simulink model "sampleModel653"  (R2023a)
settings: Solver=VariableStepAuto  StartTime=0.0  StopTime=10.0  RelTol=1e-3
undefined symbols (not defined in the file): DiscIntNeverNeededParam, magnitude, Newton, Raphson
libraries: simulink x238, slpidlib x68
(part 2 of 11)

== system sampleModel653/cfblk135 ==
  cfblk1 : Inport
  cfblk10 : Inport  Port=2
  cfblk{3,11..17} (8 alike) : Delay  SampleTime=1
  cfblk4 : slpidlib/PID Controller (2DOF)  Controller=PID  Form=Parallel  TimeDomain=Discrete-time  UseExternalTs=off  SampleTime=1  IntegratorMethod=Forward Euler  FilterMethod=Forward Euler  ControllerParametersSource=internal  P=1  I=1  UseKiTs=off  D=0  N=100  UseFilter=on  b=1  c=1  TunerSelectOption=Transfer Function Based (PID Tuner App)  InitialConditionSource=internal  InitialConditionForIntegrator=0  InitialConditionForFilter=0  DifferentiatorICPrevScaledInput=0  ExternalReset=none  TrackingMode=off  Kt=1  LimitOutput=off  SatLimitsSource=internal  UpperSaturationLimit=inf  LowerSaturationLimit=-inf  LinearizeAsGain=off  AntiWindupMode=none  Kb=1  LimitIntegrator=off  UpperIntegratorSaturationLimit=inf  LowerIntegratorSaturationLimit=-inf  POutMin=[]  POutMax=[]  IOutMin=[]  IOutMax=[]  DOutMin=[]  DOutMax=[]  NOutMin=[]  NOutMax=[]  bOutMin=[]  bOutMax=[]  cOutMin=[]  cOutMax=[]  SumOutMin=[]  SumOutMax=[]  SaturationOutMin=[]  SaturationOutMax=[]  PParamMin=[]  PParamMax=[]  IParamMin=[]  IParamMax=[]  DParamMin=[]  DParamMax=[]  NParamMin=[]  NParamMax=[]  bParamMin=[]  bParamMax=[]  cParamMin=[]  cParamMax=[]  KbParamMin=[]  KbParamMax=[]  KtParamMin=[]  KtParamMax=[]  KbOutMin=[]  KbOutMax=[]  KtOutMin=[]  KtOutMax=[]  IntegratorOutMin=[]  IntegratorOutMax=[]  FilterOutMin=[]  FilterOutMax=[]  SumI1OutMin=[]  SumI1OutMax=[]  SumI2OutMin=[]  SumI2OutMax=[]  SumI3OutMin=[]  SumI3OutMax=[]  SumI4OutMin=[]  SumI4OutMax=[]  SumDOutMin=[]  SumDOutMax=[]  Sum1OutMin=[]  Sum1OutMax=[]  Sum2OutMin=[]  Sum2OutMax=[]  Sum3OutMin=[]  Sum3OutMax=[]  DifferentiatorOutMin=[]  DifferentiatorOutMax=[]  FilterDiffOutCoefMin=[]  FilterDiffOutCoefMax=[]  ReciprocalOutMin=[]  ReciprocalOutMax=[]  SumDenOutMin=[]  SumDenOutMax=[]  SumNumOutMin=[]  SumNumOutMax=[]  DivideOutMin=[]  DivideOutMax=[]  UdiffTsProdOutMin=[]  UdiffTsProdOutMax=[]  NTsProdOutMin=[]  NTsProdOutMax=[]  UintegralTsProdOutMin=[]  UintegralTsProdOutMax=[]  UngainTsProdOutMin=[]  UngainTsProdOutMax=[]  ClampingZeroOutDataTypeStr=Inherit: Inherit via back propagation  ClampingZeroOutMin=[]  ClampingZeroOutMax=[]  FilterDenConstantOutDataTypeStr=Inherit: Inherit via back propagation  FilterDenConstantOutMin=[]  FilterDenConstantOutMax=[]  PCopyOutDataTypeStr=Inherit: Inherit via back propagation  PCopyOutMin=[]  PCopyOutMax=[]  NCopyOutDataTypeStr=Inherit: Inherit via back propagation  NCopyOutMin=[]  NCopyOutMax=[]  IntegratorContinuousStateAttributes=''  IntegratorStateMustResolveToSignalObject=off  IntegratorRTWStateStorageClass=Auto  FilterContinuousStateAttributes=''  FilterStateMustResolveToSignalObject=off  FilterRTWStateStorageClass=Auto  ParallelPVariant=InternalParameters  IdealPVariant=Disabled  IVariant=InternalParameters  DVariant=InternalParameters  bVariant=InternalParameters  cVariant=InternalParameters  IntegratorVariant=Discrete  SatVariant=Disabled  AWVariant=Passthrough  PCopyVariant=Disabled  TRVariant=Disabled  FdbkBlocksVariant=Forward  IdealPFdbkVariant=Disabled  SatFdbkVariant=Disabled  DerivativeFilterVariant=ForwardEulerFilter  NVariant=InternalParameters  NCopyVariant=Disabled  FilterICVariant=InternalICsFilter  IntegratorICVariant=InternalICs  ExternalResetVariant=Disabled  TRSumVariant=Passthrough  SumFdbkVariant=Disabled  SumVariant=Sum_PID  TsampFilterVariant=InternalTs  TsampNgainVariant=Passthrough  TsampIntegralVariant=Disabled_SignalSpec  ExternalSaturationOutDataTypeStr=Inherit: Same as second input
      settings: LibrarySourceBlock=simulink/Discrete/Discrete PID Controller (2DOF)
  cfblk5 : simulink/Discrete/Transfer Fcn Lead or Lag  PoleZ=0.95  ZeroZ=0.75  ICPrevOutput=0.0  ICPrevInput=0.0  DoSatur=off
  cfblk6 : MinMax  Inputs=3
  cfblk7 : Subsystem
  cfblk8 : Subsystem
  cfblk9 : Subsystem
  cfblk2 : Outport
  wires:
  cfblk9/1(cfblk2) -> cfblk2/1
  cfblk9/2(cfblk14) -> cfblk3/1, cfblk11/1
  cfblk10/1 -> cfblk8/2(cfblk11), cfblk9/2(cfblk12), cfblk6/3
  cfblk8/1(cfblk2) -> cfblk9/1(cfblk1), cfblk6/2
  cfblk1/1 -> cfblk4/1
  cfblk7/1(cfblk2) -> cfblk5/1, cfblk17/1
  cfblk5/1 -> cfblk15/1, cfblk16/1
  cfblk6/1 -> cfblk7/3(cfblk7), cfblk12/1, cfblk13/1, cfblk14/1
  cfblk4/1 -> cfblk8/4(cfblk13)
  cfblk3/1 -> cfblk6/1, cfblk7/2(cfblk6)
  cfblk11/1 -> cfblk8/1(cfblk1)
  cfblk12/1 -> cfblk8/3(cfblk12)
  cfblk13/1 -> cfblk9/3(cfblk13)
  cfblk14/1 -> cfblk8/5(cfblk14)
  cfblk15/1 -> cfblk4/2
  cfblk16/1 -> cfblk7/1(cfblk1)
  cfblk17/1 -> cfblk8/6(cfblk15)

== system sampleModel653/cfblk136 ==
  cfblk1 : Inport
  cfblk3 : DiscreteIntegrator  ICPrevOutput=DiscIntNeverNeededParam  ICPrevScaledInput=DiscIntNeverNeededParam
  cfblk4 : Trigonometry
  cfblk5 : Squeeze
  cfblk6 : Constant  Value=[-159954110.275562]  SampleTime=1
  cfblk7 : Subsystem
  cfblk8 : Delay  SampleTime=1
  cfblk2 : Outport
  wires:
  cfblk6/1 -> cfblk5/1
  cfblk3/1 -> cfblk2/1, cfblk8/1
  cfblk7/1(cfblk2) -> cfblk3/1
  cfblk1/1 -> cfblk7/1(cfblk1)
  cfblk5/1 -> cfblk4/1
  cfblk4/1 -> cfblk7/2(cfblk13)
  cfblk8/1 -> cfblk7/3(cfblk14)

== system sampleModel653/cfblk137 ==
  cfblk1 : Inport
  cfblk13 : Inport  Port=2
  cfblk10 : Subsystem
  cfblk11 : Subsystem
  cfblk12 : Subsystem
  cfblk15 : Delay  SampleTime=1
  cfblk16 : Delay  SampleTime=1
  cfblk17 : Delay  SampleTime=1
  cfblk3 : DiscreteTransferFcn  SampleTime=1
  cfblk4 : DiscreteStateSpace
  cfblk5 : Signum
  cfblk6 : simulink/Math Operations/MinMax Running Resettable  Function=min  vinit=0.0
  cfblk7 : Reshape
  cfblk8 : Constant  Value=[-21079559.337521]  SampleTime=1
  cfblk9 : Subsystem
  cfblk2 : Outport
  cfblk14 : Outport  Port=2
  wires:
  cfblk4/1 -> cfblk10/1(cfblk1)
  cfblk5/1 -> cfblk14/1, cfblk9/2(cfblk7)
  cfblk8/1 -> cfblk10/2(cfblk12), cfblk9/3(cfblk8)
  cfblk9/1(cfblk2) -> cfblk4/1
  cfblk7/1 -> cfblk12/1(cfblk1)
  cfblk6/1 -> cfblk5/1
  cfblk3/1 -> cfblk2/1
  cfblk1/1 -> cfblk7/1, cfblk9/4(cfblk9)
  cfblk11/1(cfblk2) -> cfblk6/2
  cfblk13/1 -> cfblk12/2(cfblk6)
  cfblk10/2(cfblk13) -> cfblk16/1, cfblk17/1
  cfblk12/1(cfblk2) -> cfblk3/1
  cfblk12/2(cfblk7) -> cfblk11/1(cfblk1)
  cfblk10/1(cfblk2) -> cfblk15/1
  cfblk15/1 -> cfblk6/1
  cfblk16/1 -> cfblk9/1(cfblk1)
  cfblk17/1 -> cfblk11/2(cfblk8)

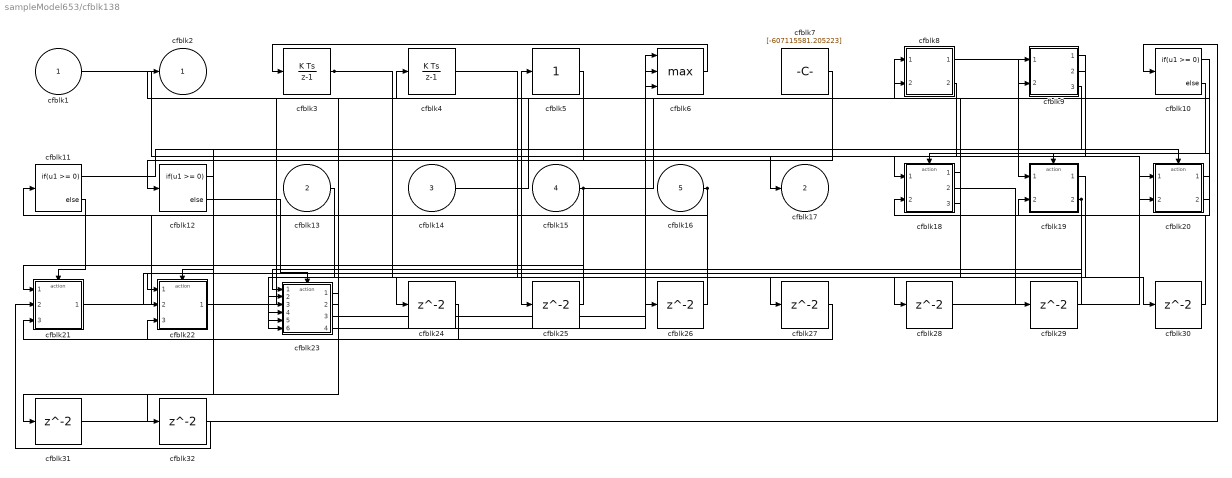
== system sampleModel653/cfblk138 ==
  cfblk1 : Inport
  cfblk13 : Inport  Port=2
  cfblk14 : Inport  Port=3
  cfblk15 : Inport  Port=4
  cfblk16 : Inport  Port=5
  cfblk10 : If  IfExpression=u1 >= 0  SampleTime=1
  cfblk11 : If  IfExpression=u1 >= 0  SampleTime=1
  cfblk12 : If  IfExpression=u1 >= 0  SampleTime=1
  cfblk18 : Subsystem  TreatAsAtomicUnit=on
  cfblk19 : Subsystem  TreatAsAtomicUnit=on
  cfblk20 : Subsystem  TreatAsAtomicUnit=on
  cfblk21 : Subsystem  TreatAsAtomicUnit=on
  cfblk22 : Subsystem  TreatAsAtomicUnit=on
  cfblk23 : Subsystem  TreatAsAtomicUnit=on
  cfblk{24..32} (9 alike) : Delay  SampleTime=1
  cfblk3 : DiscreteIntegrator  ICPrevOutput=DiscIntNeverNeededParam  ICPrevScaledInput=DiscIntNeverNeededParam
  cfblk4 : DiscreteIntegrator  ICPrevOutput=DiscIntNeverNeededParam  ICPrevScaledInput=DiscIntNeverNeededParam
  cfblk5 : simulink/Math Operations/Slider Gain  gain=1  low=0  high=2
  cfblk6 : MinMax  Function=max  Inputs=3
  cfblk7 : Constant  Value=[-607115581.205223]  SampleTime=1
  cfblk8 : Subsystem
  cfblk9 : Subsystem
  cfblk2 : Outport
  cfblk17 : Outport  Port=2
  wires:
  cfblk9/1(cfblk2) -> cfblk18/1(cfblk1)
  cfblk3/1 -> cfblk26/1, cfblk27/1
  cfblk15/1 -> cfblk8/1(cfblk1), cfblk23/4(cfblk12), cfblk9/2(cfblk12)
  cfblk7/1 -> cfblk12/1
  cfblk21/1(cfblk2) -> cfblk5/1
  cfblk1/1 -> cfblk20/2(cfblk13)
  cfblk22/1(cfblk2) -> cfblk6/1
  cfblk9/2(cfblk13) -> cfblk17/1
  cfblk18/3(cfblk9) -> cfblk4/1
  cfblk16/1 -> cfblk23/2(cfblk10), cfblk23/5(cfblk13)
  cfblk6/1 -> cfblk3/1
  cfblk14/1 -> cfblk8/2(cfblk7)
  cfblk8/1(cfblk2) -> cfblk19/1(cfblk1)
  cfblk8/2(cfblk8) -> cfblk22/1(cfblk1)
  cfblk20/1(cfblk2) -> cfblk19/2(cfblk12)
  cfblk13/1 -> cfblk23/3(cfblk11)
  cfblk19/2(cfblk13) -> cfblk22/2(cfblk7), cfblk23/6(cfblk14)
  cfblk20/2(cfblk14) -> cfblk9/1(cfblk1)
  cfblk23/2(cfblk15) -> cfblk2/1
  cfblk23/3(cfblk16) -> cfblk6/2
  cfblk23/4(cfblk17) -> cfblk6/3
  cfblk10/1 -> cfblk18/Action
  cfblk10/2 -> cfblk19/Action
  cfblk11/1 -> cfblk20/Action
  cfblk11/2 -> cfblk21/Action
  cfblk12/1 -> cfblk22/Action
  cfblk12/2 -> cfblk23/Action
  cfblk19/1(cfblk2) -> cfblk24/1
  cfblk24/1 -> cfblk21/3(cfblk12)
  cfblk5/1 -> cfblk25/1
  cfblk25/1 -> cfblk21/1(cfblk1)
  cfblk26/1 -> cfblk11/1
  cfblk27/1 -> cfblk22/3(cfblk8)
  cfblk18/1(cfblk2) -> cfblk28/1
  cfblk28/1 -> cfblk20/1(cfblk1)
  cfblk18/2(cfblk8) -> cfblk29/1
  cfblk29/1 -> cfblk23/1(cfblk1)
  cfblk4/1 -> cfblk30/1
  cfblk30/1 -> cfblk18/2(cfblk7)
  cfblk23/1(cfblk2) -> cfblk31/1
  cfblk31/1 -> cfblk10/1
  cfblk9/3(cfblk14) -> cfblk32/1
  cfblk32/1 -> cfblk21/2(cfblk11)

== system sampleModel653/cfblk139 ==
  cfblk1 : Inport
  cfblk14 : Inport  Port=2
  cfblk15 : Inport  Port=3
  cfblk10 : Subsystem
  cfblk11 : Subsystem
  cfblk12 : Subsystem
  cfblk13 : Subsystem
  cfblk{17..21} (5 alike) : Delay  SampleTime=1
  cfblk3 : PropagationDelay  SampleTime=1
  cfblk4 : DiscreteZeroPole  Poles=[0 0.5]  Gain=1
  cfblk5 : Signum
  cfblk6 : Assignment  DiagnosticForDimensions=Warning  IndexOptions=Index vector (dialog)  Indices=1  OutputSizes=1
  cfblk7 : PermuteDimensions
  cfblk8 : Abs  SaturateOnIntegerOverflow=off
  cfblk9 : Sum  Inputs=+-
  cfblk2 : Outport
  cfblk16 : Outport  Port=2
  wires:
  cfblk12/1(cfblk2) -> cfblk7/1
  cfblk15/1 -> cfblk9/1, cfblk11/6(cfblk16)
  cfblk12/2(cfblk11) -> cfblk11/1(cfblk1)
  cfblk9/1 -> cfblk2/1
  cfblk11/1(cfblk2) -> cfblk3/1
  cfblk1/1 -> cfblk5/1
  cfblk4/1 -> cfblk20/1, cfblk21/1
  cfblk3/1 -> cfblk4/1
  cfblk7/1 -> cfblk18/1, cfblk19/1
  cfblk10/1(cfblk2) -> cfblk8/1
  cfblk12/3(cfblk12) -> cfblk3/2
  cfblk5/1 -> cfblk6/2, cfblk11/3(cfblk13)
  cfblk12/4(cfblk13) -> cfblk9/2
  cfblk10/2(cfblk8) -> cfblk13/2(cfblk6)
  cfblk14/1 -> cfblk10/1(cfblk1)
  cfblk13/1(cfblk2) -> cfblk12/1(cfblk1)
  cfblk6/1 -> cfblk10/2(cfblk7), cfblk11/4(cfblk14)
  cfblk10/3(cfblk9) -> cfblk16/1, cfblk13/3(cfblk7), cfblk13/4(cfblk8)
  cfblk8/1 -> cfblk17/1
  cfblk17/1 -> cfblk6/1
  cfblk18/1 -> cfblk13/1(cfblk1)
  cfblk19/1 -> cfblk12/2(cfblk10)
  cfblk20/1 -> cfblk11/2(cfblk12)
  cfblk21/1 -> cfblk11/5(cfblk15)

== system sampleModel653/cfblk140 ==
  cfblk1 : Inport
  cfblk7 : Inport  Port=2
  cfblk8 : Inport  Port=3
  cfblk9 : Inport  Port=4
  cfblk10 : Inport  Port=5
  cfblk11 : Delay  SampleTime=1
  cfblk3 : PermuteDimensions
  cfblk4 : Subsystem
  cfblk5 : Subsystem
  cfblk6 : Subsystem
  cfblk2 : Outport
  wires:
  cfblk10/1 -> cfblk4/2(cfblk11), cfblk6/5(cfblk7)
  cfblk8/1 -> cfblk2/1
  cfblk7/1 -> cfblk5/1(cfblk1), cfblk6/2(cfblk4)
  cfblk9/1 -> cfblk4/3(cfblk12)
  cfblk1/1 -> cfblk4/4(cfblk13), cfblk6/3(cfblk5)
  cfblk5/1(cfblk2) -> cfblk3/1
  cfblk6/1(cfblk2) -> cfblk5/2(cfblk7)
  cfblk4/1(cfblk2) -> cfblk5/3(cfblk8)
  cfblk4/2(cfblk14) -> cfblk6/1(cfblk1), cfblk6/4(cfblk6)
  cfblk3/1 -> cfblk11/1
  cfblk11/1 -> cfblk4/1(cfblk1)

== system sampleModel653/cfblk141 ==
  cfblk1 : Inport
  cfblk5 : Inport  Port=2
  cfblk3 : DiscreteIntegrator  ICPrevOutput=DiscIntNeverNeededParam  ICPrevScaledInput=DiscIntNeverNeededParam
  cfblk4 : DotProduct  OutDataTypeStr=Inherit: Inherit via internal rule
  cfblk2 : Outport
  cfblk6 : Outport  Port=2
  cfblk7 : Outport  Port=3
  wires:
  cfblk5/1 -> cfblk4/1
  cfblk4/1 -> cfblk6/1, cfblk3/1
  cfblk3/1 -> cfblk2/1, cfblk7/1
  cfblk1/1 -> cfblk4/2

== system sampleModel653/cfblk142 ==
  cfblk1 : Inport
  cfblk15 : Inport  Port=2
  cfblk10 : Subsystem
  cfblk11 : Subsystem
  cfblk12 : Subsystem
  cfblk13 : Subsystem
  cfblk14 : Subsystem
  cfblk{17..21} (5 alike) : Delay  SampleTime=1
  cfblk3 : slpidlib/PID Controller (2DOF)  Controller=PID  Form=Parallel  TimeDomain=Discrete-time  UseExternalTs=off  SampleTime=1  IntegratorMethod=Forward Euler  FilterMethod=Forward Euler  ControllerParametersSource=internal  P=1  I=1  UseKiTs=off  D=0  N=100  UseFilter=on  b=1  c=1  TunerSelectOption=Transfer Function Based (PID Tuner App)  InitialConditionSource=internal  InitialConditionForIntegrator=0  InitialConditionForFilter=0  DifferentiatorICPrevScaledInput=0  ExternalReset=none  TrackingMode=off  Kt=1  LimitOutput=off  SatLimitsSource=internal  UpperSaturationLimit=inf  LowerSaturationLimit=-inf  LinearizeAsGain=off  AntiWindupMode=none  Kb=1  LimitIntegrator=off  UpperIntegratorSaturationLimit=inf  LowerIntegratorSaturationLimit=-inf  POutMin=[]  POutMax=[]  IOutMin=[]  IOutMax=[]  DOutMin=[]  DOutMax=[]  NOutMin=[]  NOutMax=[]  bOutMin=[]  bOutMax=[]  cOutMin=[]  cOutMax=[]  SumOutMin=[]  SumOutMax=[]  SaturationOutMin=[]  SaturationOutMax=[]  PParamMin=[]  PParamMax=[]  IParamMin=[]  IParamMax=[]  DParamMin=[]  DParamMax=[]  NParamMin=[]  NParamMax=[]  bParamMin=[]  bParamMax=[]  cParamMin=[]  cParamMax=[]  KbParamMin=[]  KbParamMax=[]  KtParamMin=[]  KtParamMax=[]  KbOutMin=[]  KbOutMax=[]  KtOutMin=[]  KtOutMax=[]  IntegratorOutMin=[]  IntegratorOutMax=[]  FilterOutMin=[]  FilterOutMax=[]  SumI1OutMin=[]  SumI1OutMax=[]  SumI2OutMin=[]  SumI2OutMax=[]  SumI3OutMin=[]  SumI3OutMax=[]  SumI4OutMin=[]  SumI4OutMax=[]  SumDOutMin=[]  SumDOutMax=[]  Sum1OutMin=[]  Sum1OutMax=[]  Sum2OutMin=[]  Sum2OutMax=[]  Sum3OutMin=[]  Sum3OutMax=[]  DifferentiatorOutMin=[]  DifferentiatorOutMax=[]  FilterDiffOutCoefMin=[]  FilterDiffOutCoefMax=[]  ReciprocalOutMin=[]  ReciprocalOutMax=[]  SumDenOutMin=[]  SumDenOutMax=[]  SumNumOutMin=[]  SumNumOutMax=[]  DivideOutMin=[]  DivideOutMax=[]  UdiffTsProdOutMin=[]  UdiffTsProdOutMax=[]  NTsProdOutMin=[]  NTsProdOutMax=[]  UintegralTsProdOutMin=[]  UintegralTsProdOutMax=[]  UngainTsProdOutMin=[]  UngainTsProdOutMax=[]  ClampingZeroOutDataTypeStr=Inherit: Inherit via back propagation  ClampingZeroOutMin=[]  ClampingZeroOutMax=[]  FilterDenConstantOutDataTypeStr=Inherit: Inherit via back propagation  FilterDenConstantOutMin=[]  FilterDenConstantOutMax=[]  PCopyOutDataTypeStr=Inherit: Inherit via back propagation  PCopyOutMin=[]  PCopyOutMax=[]  NCopyOutDataTypeStr=Inherit: Inherit via back propagation  NCopyOutMin=[]  NCopyOutMax=[]  IntegratorContinuousStateAttributes=''  IntegratorStateMustResolveToSignalObject=off  IntegratorRTWStateStorageClass=Auto  FilterContinuousStateAttributes=''  FilterStateMustResolveToSignalObject=off  FilterRTWStateStorageClass=Auto  ParallelPVariant=InternalParameters  IdealPVariant=Disabled  IVariant=InternalParameters  DVariant=InternalParameters  bVariant=InternalParameters  cVariant=InternalParameters  IntegratorVariant=Discrete  SatVariant=Disabled  AWVariant=Passthrough  PCopyVariant=Disabled  TRVariant=Disabled  FdbkBlocksVariant=Forward  IdealPFdbkVariant=Disabled  SatFdbkVariant=Disabled  DerivativeFilterVariant=ForwardEulerFilter  NVariant=InternalParameters  NCopyVariant=Disabled  FilterICVariant=InternalICsFilter  IntegratorICVariant=InternalICs  ExternalResetVariant=Disabled  TRSumVariant=Passthrough  SumFdbkVariant=Disabled  SumVariant=Sum_PID  TsampFilterVariant=InternalTs  TsampNgainVariant=Passthrough  TsampIntegralVariant=Disabled_SignalSpec  ExternalSaturationOutDataTypeStr=Inherit: Same as second input
      settings: LibrarySourceBlock=simulink/Discrete/Discrete PID Controller (2DOF)
  cfblk4 : DiscreteTransferFcn  SampleTime=1
  cfblk5 : Sqrt  Operator=rSqrt  AlgorithmType=Newton-Raphson
  cfblk6 : Reshape
  cfblk7 : Squeeze
  cfblk8 : Constant  Value=[687668237.338755]  SampleTime=1
  cfblk9 : Constant  Value=[-134938551.246694]  SampleTime=1
  cfblk2 : Outport
  cfblk16 : Outport  Port=2
  wires:
  cfblk11/1(cfblk2) -> cfblk5/1
  cfblk6/1 -> cfblk16/1
  cfblk15/1 -> cfblk3/1, cfblk13/5(cfblk12)
  cfblk14/1(cfblk2) -> cfblk11/1(cfblk1), cfblk11/3(cfblk12), cfblk18/1, cfblk19/1
  cfblk7/1 -> cfblk3/2
  cfblk9/1 -> cfblk14/1(cfblk1), cfblk12/5(cfblk11)
  cfblk13/1(cfblk2) -> cfblk2/1
  cfblk3/1 -> cfblk14/2(cfblk13), cfblk20/1
  cfblk1/1 -> cfblk6/1, cfblk13/3(cfblk10)
  cfblk8/1 -> cfblk13/2(cfblk9)
  cfblk13/2(cfblk13) -> cfblk10/1(cfblk1), cfblk11/4(cfblk13)
  cfblk10/1(cfblk2) -> cfblk12/1(cfblk1)
  cfblk12/1(cfblk2) -> cfblk14/3(cfblk14)
  cfblk10/2(cfblk11) -> cfblk12/2(cfblk8), cfblk14/5(cfblk16)
  cfblk12/2(cfblk12) -> cfblk14/4(cfblk15)
  cfblk12/3(cfblk13) -> cfblk11/2(cfblk11)
  cfblk12/4(cfblk14) -> cfblk4/1, cfblk21/1
  cfblk4/1 -> cfblk7/1
  cfblk5/1 -> cfblk17/1
  cfblk17/1 -> cfblk13/1(cfblk1)
  cfblk18/1 -> cfblk10/2(cfblk10)
  cfblk19/1 -> cfblk12/3(cfblk9)
  cfblk20/1 -> cfblk12/4(cfblk10)
  cfblk21/1 -> cfblk13/4(cfblk11)

== system sampleModel653/cfblk143 ==
  cfblk1 : Inport
  cfblk10 : Subsystem
  cfblk11 : Delay  SampleTime=1
  cfblk12 : Delay  SampleTime=1
  cfblk13 : Delay  SampleTime=1
  cfblk3 : simulink/Discrete/Difference  ICPrevInput=0.0  OutMin=[]  OutMax=[]  OutDataTypeStr=Inherit: Inherit via back propagation  OutDataType=fixdt(1, 16)  OutScaling=2^-10  DoSatur=off
  cfblk4 : simulink/Discrete/Transfer Fcn First Order  PoleZ=0.95  ICPrevOutput=0.0  DoSatur=off
  cfblk5 : simulink/Discrete/Difference  ICPrevInput=0.0  OutMin=[]  OutMax=[]  OutDataTypeStr=Inherit: Inherit via back propagation  OutDataType=fixdt(1, 16)  OutScaling=2^-10  DoSatur=off
  cfblk6 : Gain  Gain=[-693180009.173398]
  cfblk7 : UnaryMinus
  cfblk8 : Subsystem
  cfblk9 : Subsystem
  cfblk2 : Outport
  wires:
  cfblk4/1 -> cfblk10/1(cfblk1)
  cfblk3/1 -> cfblk7/1
  cfblk7/1 -> cfblk5/1
  cfblk6/1 -> cfblk2/1, cfblk8/2(cfblk8)
  cfblk10/1(cfblk2) -> cfblk9/1(cfblk1)
  cfblk1/1 -> cfblk6/1
  cfblk8/1(cfblk2) -> cfblk3/1
  cfblk5/1 -> cfblk11/1
  cfblk11/1 -> cfblk8/1(cfblk1)
  cfblk9/1(cfblk2) -> cfblk12/1
  cfblk12/1 -> cfblk4/1
  cfblk9/2(cfblk7) -> cfblk13/1
  cfblk13/1 -> cfblk10/2(cfblk8)

== system sampleModel653/cfblk144 ==
  cfblk1 : Inport
  cfblk7 : Inport  Port=2
  cfblk3 : ComplexToRealImag
  cfblk4 : Sqrt
  cfblk5 : Subsystem
  cfblk6 : Subsystem
  cfblk9 : Delay  SampleTime=1
  cfblk2 : Outport
  cfblk8 : Outport  Port=2
  wires:
  cfblk3/1 -> cfblk6/1(cfblk1)
  cfblk5/1(cfblk2) -> cfblk6/2(cfblk8), cfblk9/1
  cfblk4/1 -> cfblk5/1(cfblk1)
  cfblk3/2 -> cfblk4/1, cfblk5/3(cfblk7)
  cfblk7/1 -> cfblk5/2(cfblk6)
  cfblk1/1 -> cfblk8/1
  cfblk6/1(cfblk2) -> cfblk2/1
  cfblk9/1 -> cfblk3/1

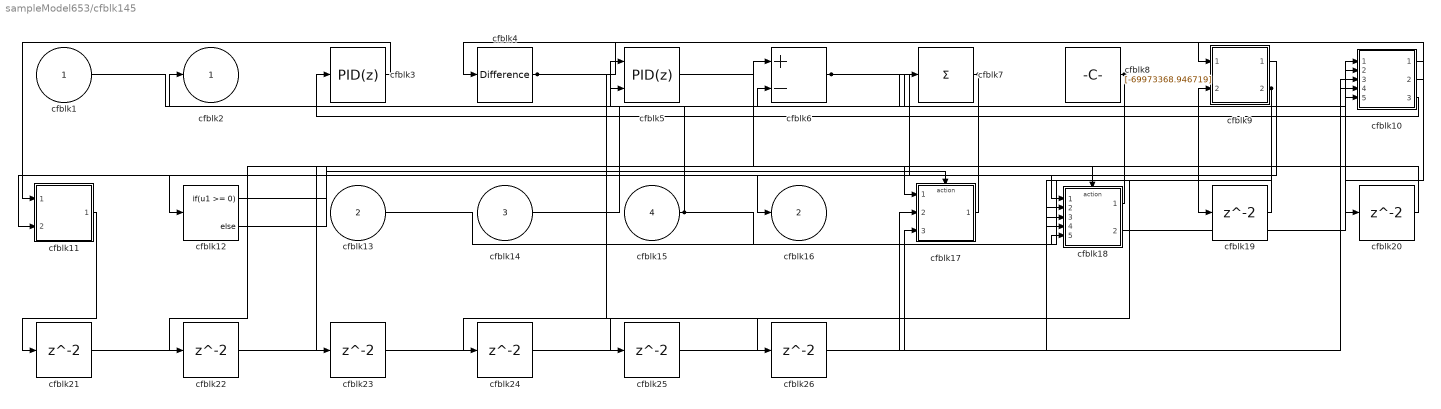
== system sampleModel653/cfblk145 ==
  cfblk1 : Inport
  cfblk13 : Inport  Port=2
  cfblk14 : Inport  Port=3
  cfblk15 : Inport  Port=4
  cfblk10 : Subsystem
  cfblk11 : Subsystem
  cfblk12 : If  IfExpression=u1 >= 0  SampleTime=1
  cfblk17 : Subsystem  TreatAsAtomicUnit=on
  cfblk18 : Subsystem  TreatAsAtomicUnit=on
  cfblk{19..26} (8 alike) : Delay  SampleTime=1
  cfblk3 : slpidlib/PID Controller  Controller=PID  Form=Parallel  TimeDomain=Discrete-time  UseExternalTs=off  SampleTime=1  IntegratorMethod=Forward Euler  FilterMethod=Forward Euler  ControllerParametersSource=internal  P=1  I=1  UseKiTs=off  D=0  N=100  UseFilter=on  TunerSelectOption=Transfer Function Based (PID Tuner App)  InitialConditionSource=internal  InitialConditionForIntegrator=0  InitialConditionForFilter=0  DifferentiatorICPrevScaledInput=0  ExternalReset=none  TrackingMode=off  Kt=1  LimitOutput=off  SatLimitsSource=internal  UpperSaturationLimit=inf  LowerSaturationLimit=-inf  LinearizeAsGain=off  AntiWindupMode=none  Kb=1  LimitIntegrator=off  UpperIntegratorSaturationLimit=inf  LowerIntegratorSaturationLimit=-inf  POutMin=[]  POutMax=[]  IOutMin=[]  IOutMax=[]  DOutMin=[]  DOutMax=[]  NOutMin=[]  NOutMax=[]  SumOutMin=[]  SumOutMax=[]  SaturationOutMin=[]  SaturationOutMax=[]  PParamMin=[]  PParamMax=[]  IParamMin=[]  IParamMax=[]  DParamMin=[]  DParamMax=[]  NParamMin=[]  NParamMax=[]  KbParamMin=[]  KbParamMax=[]  KtParamMin=[]  KtParamMax=[]  KbOutMin=[]  KbOutMax=[]  KtOutMin=[]  KtOutMax=[]  IntegratorOutMin=[]  IntegratorOutMax=[]  FilterOutMin=[]  FilterOutMax=[]  SumI1OutMin=[]  SumI1OutMax=[]  SumI2OutMin=[]  SumI2OutMax=[]  SumI3OutMin=[]  SumI3OutMax=[]  SumI4OutMin=[]  SumI4OutMax=[]  SumDOutMin=[]  SumDOutMax=[]  DifferentiatorOutMin=[]  DifferentiatorOutMax=[]  FilterDiffOutCoefMin=[]  FilterDiffOutCoefMax=[]  ReciprocalOutMin=[]  ReciprocalOutMax=[]  SumDenOutMin=[]  SumDenOutMax=[]  SumNumOutMin=[]  SumNumOutMax=[]  DivideOutMin=[]  DivideOutMax=[]  UdiffTsProdOutMin=[]  UdiffTsProdOutMax=[]  NTsProdOutMin=[]  NTsProdOutMax=[]  UintegralTsProdOutMin=[]  UintegralTsProdOutMax=[]  UngainTsProdOutMin=[]  UngainTsProdOutMax=[]  ClampingZeroOutDataTypeStr=Inherit: Inherit via back propagation  ClampingZeroOutMin=[]  ClampingZeroOutMax=[]  FilterDenConstantOutDataTypeStr=Inherit: Inherit via back propagation  FilterDenConstantOutMin=[]  FilterDenConstantOutMax=[]  PCopyOutDataTypeStr=Inherit: Inherit via back propagation  PCopyOutMin=[]  PCopyOutMax=[]  NCopyOutDataTypeStr=Inherit: Inherit via back propagation  NCopyOutMin=[]  NCopyOutMax=[]  IntegratorContinuousStateAttributes=''  IntegratorStateMustResolveToSignalObject=off  IntegratorRTWStateStorageClass=Auto  FilterContinuousStateAttributes=''  FilterStateMustResolveToSignalObject=off  FilterRTWStateStorageClass=Auto  ParallelPVariant=InternalParameters  IdealPVariant=Disabled  IVariant=InternalParameters  DVariant=InternalParameters  IntegratorVariant=Discrete  SatVariant=Disabled  AWVariant=Passthrough  PCopyVariant=Disabled  TRVariant=Disabled  FdbkBlocksVariant=Forward  IdealPFdbkVariant=Disabled  SatFdbkVariant=Disabled  DerivativeFilterVariant=ForwardEulerFilter  NVariant=InternalParameters  NCopyVariant=Disabled  FilterICVariant=InternalICsFilter  IntegratorICVariant=InternalICs  ExternalResetVariant=Disabled  TRSumVariant=Passthrough  SumFdbkVariant=Disabled  SumVariant=Sum_PID  TsampFilterVariant=InternalTs  TsampNgainVariant=Passthrough  TsampIntegralVariant=Disabled_SignalSpec  ExternalSaturationOutDataTypeStr=Inherit: Same as second input
      settings: LibrarySourceBlock=simulink/Discrete/Discrete PID Controller
  cfblk4 : simulink/Discrete/Difference  ICPrevInput=0.0  OutMin=[]  OutMax=[]  OutDataTypeStr=Inherit: Inherit via back propagation  OutDataType=fixdt(1, 16)  OutScaling=2^-10  DoSatur=off
  cfblk5 : slpidlib/PID Controller (2DOF)  Controller=PID  Form=Parallel  TimeDomain=Discrete-time  UseExternalTs=off  SampleTime=1  IntegratorMethod=Forward Euler  FilterMethod=Forward Euler  ControllerParametersSource=internal  P=1  I=1  UseKiTs=off  D=0  N=100  UseFilter=on  b=1  c=1  TunerSelectOption=Transfer Function Based (PID Tuner App)  InitialConditionSource=internal  InitialConditionForIntegrator=0  InitialConditionForFilter=0  DifferentiatorICPrevScaledInput=0  ExternalReset=none  TrackingMode=off  Kt=1  LimitOutput=off  SatLimitsSource=internal  UpperSaturationLimit=inf  LowerSaturationLimit=-inf  LinearizeAsGain=off  AntiWindupMode=none  Kb=1  LimitIntegrator=off  UpperIntegratorSaturationLimit=inf  LowerIntegratorSaturationLimit=-inf  POutMin=[]  POutMax=[]  IOutMin=[]  IOutMax=[]  DOutMin=[]  DOutMax=[]  NOutMin=[]  NOutMax=[]  bOutMin=[]  bOutMax=[]  cOutMin=[]  cOutMax=[]  SumOutMin=[]  SumOutMax=[]  SaturationOutMin=[]  SaturationOutMax=[]  PParamMin=[]  PParamMax=[]  IParamMin=[]  IParamMax=[]  DParamMin=[]  DParamMax=[]  NParamMin=[]  NParamMax=[]  bParamMin=[]  bParamMax=[]  cParamMin=[]  cParamMax=[]  KbParamMin=[]  KbParamMax=[]  KtParamMin=[]  KtParamMax=[]  KbOutMin=[]  KbOutMax=[]  KtOutMin=[]  KtOutMax=[]  IntegratorOutMin=[]  IntegratorOutMax=[]  FilterOutMin=[]  FilterOutMax=[]  SumI1OutMin=[]  SumI1OutMax=[]  SumI2OutMin=[]  SumI2OutMax=[]  SumI3OutMin=[]  SumI3OutMax=[]  SumI4OutMin=[]  SumI4OutMax=[]  SumDOutMin=[]  SumDOutMax=[]  Sum1OutMin=[]  Sum1OutMax=[]  Sum2OutMin=[]  Sum2OutMax=[]  Sum3OutMin=[]  Sum3OutMax=[]  DifferentiatorOutMin=[]  DifferentiatorOutMax=[]  FilterDiffOutCoefMin=[]  FilterDiffOutCoefMax=[]  ReciprocalOutMin=[]  ReciprocalOutMax=[]  SumDenOutMin=[]  SumDenOutMax=[]  SumNumOutMin=[]  SumNumOutMax=[]  DivideOutMin=[]  DivideOutMax=[]  UdiffTsProdOutMin=[]  UdiffTsProdOutMax=[]  NTsProdOutMin=[]  NTsProdOutMax=[]  UintegralTsProdOutMin=[]  UintegralTsProdOutMax=[]  UngainTsProdOutMin=[]  UngainTsProdOutMax=[]  ClampingZeroOutDataTypeStr=Inherit: Inherit via back propagation  ClampingZeroOutMin=[]  ClampingZeroOutMax=[]  FilterDenConstantOutDataTypeStr=Inherit: Inherit via back propagation  FilterDenConstantOutMin=[]  FilterDenConstantOutMax=[]  PCopyOutDataTypeStr=Inherit: Inherit via back propagation  PCopyOutMin=[]  PCopyOutMax=[]  NCopyOutDataTypeStr=Inherit: Inherit via back propagation  NCopyOutMin=[]  NCopyOutMax=[]  IntegratorContinuousStateAttributes=''  IntegratorStateMustResolveToSignalObject=off  IntegratorRTWStateStorageClass=Auto  FilterContinuousStateAttributes=''  FilterStateMustResolveToSignalObject=off  FilterRTWStateStorageClass=Auto  ParallelPVariant=InternalParameters  IdealPVariant=Disabled  IVariant=InternalParameters  DVariant=InternalParameters  bVariant=InternalParameters  cVariant=InternalParameters  IntegratorVariant=Discrete  SatVariant=Disabled  AWVariant=Passthrough  PCopyVariant=Disabled  TRVariant=Disabled  FdbkBlocksVariant=Forward  IdealPFdbkVariant=Disabled  SatFdbkVariant=Disabled  DerivativeFilterVariant=ForwardEulerFilter  NVariant=InternalParameters  NCopyVariant=Disabled  FilterICVariant=InternalICsFilter  IntegratorICVariant=InternalICs  ExternalResetVariant=Disabled  TRSumVariant=Passthrough  SumFdbkVariant=Disabled  SumVariant=Sum_PID  TsampFilterVariant=InternalTs  TsampNgainVariant=Passthrough  TsampIntegralVariant=Disabled_SignalSpec  ExternalSaturationOutDataTypeStr=Inherit: Same as second input
      settings: LibrarySourceBlock=simulink/Discrete/Discrete PID Controller (2DOF)
  cfblk6 : Sum  Inputs=+-
  cfblk7 : Sum  Inputs=+
  cfblk8 : Constant  Value=[-69973368.946719]  SampleTime=1
  cfblk9 : Subsystem
  cfblk2 : Outport
  cfblk16 : Outport  Port=2
  wires:
  cfblk8/1 -> cfblk12/1, cfblk18/3(cfblk11)
  cfblk4/1 -> cfblk9/1(cfblk1), cfblk26/1
  cfblk13/1 -> cfblk9/2(cfblk13)
  cfblk14/1 -> cfblk10/1(cfblk1)
  cfblk18/1(cfblk2) -> cfblk5/1
  cfblk6/1 -> cfblk18/1(cfblk1), cfblk10/5(cfblk15)
  cfblk9/1(cfblk2) -> cfblk16/1
  cfblk15/1 -> cfblk2/1, cfblk18/5(cfblk13)
  cfblk3/1 -> cfblk11/1(cfblk1)
  cfblk1/1 -> cfblk6/2
  cfblk7/1 -> cfblk11/2(cfblk7), cfblk5/2, cfblk22/1, cfblk23/1
  cfblk17/1(cfblk2) -> cfblk7/1
  cfblk18/2(cfblk14) -> cfblk10/2(cfblk12)
  cfblk10/2(cfblk16) -> cfblk4/1
  cfblk9/2(cfblk14) -> cfblk24/1, cfblk25/1
  cfblk10/3(cfblk17) -> cfblk3/1
  cfblk12/1 -> cfblk17/Action
  cfblk12/2 -> cfblk18/Action
  cfblk5/1 -> cfblk19/1
  cfblk19/1 -> cfblk6/1
  cfblk10/1(cfblk2) -> cfblk20/1
  cfblk20/1 -> cfblk17/1(cfblk1)
  cfblk11/1(cfblk2) -> cfblk21/1
  cfblk21/1 -> cfblk17/2(cfblk8)
  cfblk22/1 -> cfblk18/2(cfblk10)
  cfblk23/1 -> cfblk17/3(cfblk9)
  cfblk24/1 -> cfblk10/3(cfblk13)
  cfblk25/1 -> cfblk18/4(cfblk12)
  cfblk26/1 -> cfblk10/4(cfblk14)

== system sampleModel653/cfblk146 ==
  cfblk1 : Inport
  cfblk9 : Inport  Port=2
  cfblk10 : Inport  Port=3
  cfblk11 : Inport  Port=4
  cfblk12 : Inport  Port=5
  cfblk15 : Delay  SampleTime=1
  cfblk16 : Delay  SampleTime=1
  cfblk3 : DiscreteFilter  SampleTime=1
  cfblk4 : DotProduct  OutDataTypeStr=Inherit: Inherit via internal rule
  cfblk5 : Constant  Value=[625665338.084405]  SampleTime=1
  cfblk6 : Subsystem
  cfblk7 : Subsystem
  cfblk8 : Subsystem
  cfblk2 : Outport
  cfblk13 : Outport  Port=2
  cfblk14 : Outport  Port=3
  wires:
  cfblk4/1 -> cfblk7/1(cfblk1)
  cfblk3/1 -> cfblk2/1
  cfblk12/1 -> cfblk14/1
  cfblk9/1 -> cfblk7/2(cfblk11)
  cfblk11/1 -> cfblk6/1(cfblk1)
  cfblk8/1(cfblk2) -> cfblk7/3(cfblk12)
  cfblk1/1 -> cfblk6/2(cfblk9)
  cfblk6/1(cfblk2) -> cfblk8/1(cfblk1)
  cfblk8/2(cfblk15) -> cfblk3/1
  cfblk8/3(cfblk16) -> cfblk13/1
  cfblk10/1 -> cfblk8/4(cfblk13)
  cfblk5/1 -> cfblk8/5(cfblk14)
  cfblk6/2(cfblk10) -> cfblk4/1
  cfblk8/4(cfblk17) -> cfblk4/2
  cfblk7/1(cfblk2) -> cfblk15/1
  cfblk15/1 -> cfblk8/2(cfblk11)
  cfblk7/2(cfblk13) -> cfblk16/1
  cfblk16/1 -> cfblk8/3(cfblk12)

== system sampleModel653/cfblk147 ==
  cfblk1 : Inport
  cfblk14 : Inport  Port=2
  cfblk10 : simulink/Math Operations/MinMax Running Resettable  Function=min  vinit=0.0
  cfblk11 : Subsystem
  cfblk12 : Subsystem
  cfblk13 : Subsystem
  cfblk{15..21} (7 alike) : Delay  SampleTime=1
  cfblk3 : PropagationDelay  SampleTime=1
  cfblk4 : simulink/Discrete/Transfer Fcn Real Zero  ZeroZ=0.75  ICPrevInput=0.0  DoSatur=off
  cfblk5 : DiscreteStateSpace
  cfblk6 : DiscreteFir  SampleTime=1
  cfblk7 : slpidlib/PID Controller  Controller=PID  Form=Parallel  TimeDomain=Discrete-time  UseExternalTs=off  SampleTime=1  IntegratorMethod=Forward Euler  FilterMethod=Forward Euler  ControllerParametersSource=internal  P=1  I=1  UseKiTs=off  D=0  N=100  UseFilter=on  TunerSelectOption=Transfer Function Based (PID Tuner App)  InitialConditionSource=internal  InitialConditionForIntegrator=0  InitialConditionForFilter=0  DifferentiatorICPrevScaledInput=0  ExternalReset=none  TrackingMode=off  Kt=1  LimitOutput=off  SatLimitsSource=internal  UpperSaturationLimit=inf  LowerSaturationLimit=-inf  LinearizeAsGain=off  AntiWindupMode=none  Kb=1  LimitIntegrator=off  UpperIntegratorSaturationLimit=inf  LowerIntegratorSaturationLimit=-inf  POutMin=[]  POutMax=[]  IOutMin=[]  IOutMax=[]  DOutMin=[]  DOutMax=[]  NOutMin=[]  NOutMax=[]  SumOutMin=[]  SumOutMax=[]  SaturationOutMin=[]  SaturationOutMax=[]  PParamMin=[]  PParamMax=[]  IParamMin=[]  IParamMax=[]  DParamMin=[]  DParamMax=[]  NParamMin=[]  NParamMax=[]  KbParamMin=[]  KbParamMax=[]  KtParamMin=[]  KtParamMax=[]  KbOutMin=[]  KbOutMax=[]  KtOutMin=[]  KtOutMax=[]  IntegratorOutMin=[]  IntegratorOutMax=[]  FilterOutMin=[]  FilterOutMax=[]  SumI1OutMin=[]  SumI1OutMax=[]  SumI2OutMin=[]  SumI2OutMax=[]  SumI3OutMin=[]  SumI3OutMax=[]  SumI4OutMin=[]  SumI4OutMax=[]  SumDOutMin=[]  SumDOutMax=[]  DifferentiatorOutMin=[]  DifferentiatorOutMax=[]  FilterDiffOutCoefMin=[]  FilterDiffOutCoefMax=[]  ReciprocalOutMin=[]  ReciprocalOutMax=[]  SumDenOutMin=[]  SumDenOutMax=[]  SumNumOutMin=[]  SumNumOutMax=[]  DivideOutMin=[]  DivideOutMax=[]  UdiffTsProdOutMin=[]  UdiffTsProdOutMax=[]  NTsProdOutMin=[]  NTsProdOutMax=[]  UintegralTsProdOutMin=[]  UintegralTsProdOutMax=[]  UngainTsProdOutMin=[]  UngainTsProdOutMax=[]  ClampingZeroOutDataTypeStr=Inherit: Inherit via back propagation  ClampingZeroOutMin=[]  ClampingZeroOutMax=[]  FilterDenConstantOutDataTypeStr=Inherit: Inherit via back propagation  FilterDenConstantOutMin=[]  FilterDenConstantOutMax=[]  PCopyOutDataTypeStr=Inherit: Inherit via back propagation  PCopyOutMin=[]  PCopyOutMax=[]  NCopyOutDataTypeStr=Inherit: Inherit via back propagation  NCopyOutMin=[]  NCopyOutMax=[]  IntegratorContinuousStateAttributes=''  IntegratorStateMustResolveToSignalObject=off  IntegratorRTWStateStorageClass=Auto  FilterContinuousStateAttributes=''  FilterStateMustResolveToSignalObject=off  FilterRTWStateStorageClass=Auto  ParallelPVariant=InternalParameters  IdealPVariant=Disabled  IVariant=InternalParameters  DVariant=InternalParameters  IntegratorVariant=Discrete  SatVariant=Disabled  AWVariant=Passthrough  PCopyVariant=Disabled  TRVariant=Disabled  FdbkBlocksVariant=Forward  IdealPFdbkVariant=Disabled  SatFdbkVariant=Disabled  DerivativeFilterVariant=ForwardEulerFilter  NVariant=InternalParameters  NCopyVariant=Disabled  FilterICVariant=InternalICsFilter  IntegratorICVariant=InternalICs  ExternalResetVariant=Disabled  TRSumVariant=Passthrough  SumFdbkVariant=Disabled  SumVariant=Sum_PID  TsampFilterVariant=InternalTs  TsampNgainVariant=Passthrough  TsampIntegralVariant=Disabled_SignalSpec  ExternalSaturationOutDataTypeStr=Inherit: Same as second input
      settings: LibrarySourceBlock=simulink/Discrete/Discrete PID Controller
  cfblk8 : simulink/Discrete/Difference  ICPrevInput=0.0  OutMin=[]  OutMax=[]  OutDataTypeStr=Inherit: Inherit via back propagation  OutDataType=fixdt(1, 16)  OutScaling=2^-10  DoSatur=off
  cfblk9 : Product
  cfblk2 : Outport
  wires:
  cfblk12/1(cfblk2) -> cfblk6/1
  cfblk11/1(cfblk2) -> cfblk5/1
  cfblk7/1 -> cfblk9/1, cfblk11/3(cfblk6)
  cfblk13/1(cfblk2) -> cfblk4/1
  cfblk1/1 -> cfblk7/1
  cfblk10/1 -> cfblk12/1(cfblk1)
  cfblk4/1 -> cfblk3/2
  cfblk12/2(cfblk14) -> cfblk13/2(cfblk6)
  cfblk13/2(cfblk7) -> cfblk8/1
  cfblk14/1 -> cfblk9/2
  cfblk3/1 -> cfblk11/2(cfblk5), cfblk11/4(cfblk7), cfblk16/1
  cfblk13/3(cfblk8) -> cfblk11/1(cfblk1)
  cfblk9/1 -> cfblk10/2
  cfblk13/4(cfblk9) -> cfblk2/1
  cfblk13/5(cfblk10) -> cfblk20/1, cfblk21/1
  cfblk6/1 -> cfblk15/1
  cfblk15/1 -> cfblk10/1
  cfblk16/1 -> cfblk12/3(cfblk11)
  cfblk5/1 -> cfblk17/1
  cfblk17/1 -> cfblk3/1
  cfblk11/2(cfblk8) -> cfblk18/1
  cfblk18/1 -> cfblk13/1(cfblk1)
  cfblk8/1 -> cfblk19/1
  cfblk19/1 -> cfblk12/2(cfblk10)
  cfblk20/1 -> cfblk12/4(cfblk12)
  cfblk21/1 -> cfblk12/5(cfblk13)

== system sampleModel653/cfblk148 ==
  cfblk1 : Inport
  cfblk6 : Inport  Port=2
  cfblk7 : Inport  Port=3
  cfblk8 : Inport  Port=4
  cfblk3 : Constant  Value=[726432575.877130]  SampleTime=1
  cfblk4 : Subsystem
  cfblk5 : Subsystem
  cfblk2 : Outport
  wires:
  cfblk6/1 -> cfblk4/1(cfblk1)
  cfblk1/1 -> cfblk5/1(cfblk1)
  cfblk3/1 -> cfblk2/1

== system sampleModel653/cfblk149 ==
  cfblk1 : Inport
  cfblk15 : Inport  Port=2
  cfblk10 : Subsystem
  cfblk11 : Subsystem
  cfblk12 : Subsystem
  cfblk13 : Subsystem
  cfblk14 : Subsystem
  cfblk{16..22} (7 alike) : Delay  SampleTime=1
  cfblk3 : PropagationDelay  SampleTime=1
  cfblk4 : DiscreteFilter  SampleTime=1
  cfblk5 : Sum  Inputs=+
  cfblk6 : ComplexToMagnitudeAngle
  cfblk7 : DotProduct  OutDataTypeStr=Inherit: Inherit via internal rule
  cfblk8 : Trigonometry
  cfblk9 : Subsystem
  cfblk2 : Outport
  wires:
  cfblk1/1 -> cfblk5/1
  cfblk3/1 -> cfblk2/1
  cfblk13/1(cfblk2) -> cfblk11/1(cfblk1)
  cfblk7/1 -> cfblk9/1(cfblk1)
  cfblk6/2 -> cfblk3/1, cfblk18/1
  cfblk15/1 -> cfblk8/1
  cfblk8/1 -> cfblk12/1(cfblk1)
  cfblk10/1(cfblk2) -> cfblk12/2(cfblk5), cfblk20/1
  cfblk12/1(cfblk2) -> cfblk3/2
  cfblk12/2(cfblk6) -> cfblk7/1
  cfblk5/1 -> cfblk4/1
  cfblk12/3(cfblk7) -> cfblk6/1
  cfblk4/1 -> cfblk13/1(cfblk1)
  cfblk14/1(cfblk2) -> cfblk10/2(cfblk10)
  cfblk11/1(cfblk2) -> cfblk14/2(cfblk9)
  cfblk11/2(cfblk7) -> cfblk7/2, cfblk22/1
  cfblk9/1(cfblk2) -> cfblk16/1
  cfblk16/1 -> cfblk14/1(cfblk1)
  cfblk6/1 -> cfblk17/1
  cfblk17/1 -> cfblk11/2(cfblk6)
  cfblk18/1 -> cfblk13/4(cfblk11)
  cfblk12/4(cfblk8) -> cfblk19/1
  cfblk19/1 -> cfblk10/1(cfblk1)
  cfblk20/1 -> cfblk14/3(cfblk10)
  cfblk14/2(cfblk11) -> cfblk21/1
  cfblk21/1 -> cfblk13/2(cfblk9)
  cfblk22/1 -> cfblk13/3(cfblk10)

== system sampleModel653/cfblk150 ==
  cfblk1 : Inport
  cfblk10 : Delay  SampleTime=1
  cfblk3 : simulink/Discrete/Difference  ICPrevInput=0.0  OutMin=[]  OutMax=[]  OutDataTypeStr=Inherit: Inherit via back propagation  OutDataType=fixdt(1, 16)  OutScaling=2^-10  DoSatur=off
  cfblk4 : Squeeze
  cfblk5 : Sum  Inputs=|++
  cfblk6 : Constant  Value=[-875012264.866735]  SampleTime=1
  cfblk7 : Subsystem
  cfblk8 : Subsystem
  cfblk9 : Delay  SampleTime=1
  cfblk2 : Outport
  wires:
  cfblk1/1 -> cfblk7/1(cfblk1)
  cfblk7/1(cfblk2) -> cfblk4/1
  cfblk8/1(cfblk2) -> cfblk3/1
  cfblk4/1 -> cfblk8/1(cfblk1), cfblk5/1
  cfblk7/2(cfblk10) -> cfblk2/1, cfblk8/3(cfblk8), cfblk5/2
  cfblk6/1 -> cfblk8/2(cfblk7)
  cfblk3/1 -> cfblk9/1
  cfblk9/1 -> cfblk7/2(cfblk8)
  cfblk5/1 -> cfblk10/1
  cfblk10/1 -> cfblk7/3(cfblk9)

== system sampleModel653/cfblk151 ==
  cfblk1 : Inport
  cfblk10 : Inport  Port=2
  cfblk11 : Inport  Port=3
  cfblk12 : Delay  SampleTime=1
  cfblk13 : Delay  SampleTime=1
  cfblk14 : Delay  SampleTime=1
  cfblk3 : Gain  Gain=[-249221804.491329]
  cfblk4 : ComplexToMagnitudeAngle
  cfblk5 : simulink/Math Operations/MinMax Running Resettable  Function=min  vinit=0.0
  cfblk6 : Constant  Value=[-204190769.937497]  SampleTime=1
  cfblk7 : Subsystem
  cfblk8 : Subsystem
  cfblk9 : Subsystem
  cfblk2 : Outport
  wires:
  cfblk9/1(cfblk2) -> cfblk5/1, cfblk7/3(cfblk13)
  cfblk6/1 -> cfblk4/1
  cfblk1/1 -> cfblk9/1(cfblk1), cfblk7/2(cfblk12)
  cfblk4/1 -> cfblk8/1(cfblk1)
  cfblk3/1 -> cfblk7/1(cfblk1), cfblk2/1
  cfblk4/2 -> cfblk8/2(cfblk9)
  cfblk5/1 -> cfblk7/4(cfblk14), cfblk12/1
  cfblk11/1 -> cfblk3/1, cfblk9/6(cfblk13)
  cfblk8/1(cfblk2) -> cfblk5/2
  cfblk10/1 -> cfblk8/3(cfblk10)
  cfblk8/2(cfblk11) -> cfblk9/5(cfblk12)
  cfblk12/1 -> cfblk9/2(cfblk9)
  cfblk7/1(cfblk2) -> cfblk13/1
  cfblk13/1 -> cfblk9/3(cfblk10)
  cfblk7/2(cfblk15) -> cfblk14/1
  cfblk14/1 -> cfblk9/4(cfblk11)

== system sampleModel653/cfblk152 ==
  cfblk1 : Inport
  cfblk13 : Inport  Port=2
  cfblk10 : Subsystem
  cfblk11 : Subsystem
  cfblk12 : Subsystem
  cfblk{15..19} (5 alike) : Delay  SampleTime=1
  cfblk3 : Delay  DelayLengthSource=Input port  SampleTime=1
      settings: InputPortMap=u0,p1
  cfblk4 : Sqrt
  cfblk5 : Sin  TimeSource=Use external signal  SampleTime=0
  cfblk6 : MinMax  Function=max  Inputs=3
  cfblk7 : Constant  Value=[-957673549.399829]  SampleTime=1
  cfblk8 : Constant  Value=[-668192992.482745]  SampleTime=1
  cfblk9 : Subsystem
  cfblk2 : Outport
  cfblk14 : Outport  Port=2
  wires:
  cfblk12/1(cfblk2) -> cfblk4/1
  cfblk10/1(cfblk2) -> cfblk14/1, cfblk11/5(cfblk13)
  cfblk12/2(cfblk13) -> cfblk9/1(cfblk1)
  cfblk8/1 -> cfblk2/1, cfblk10/2(cfblk6)
  cfblk7/1 -> cfblk5/1, cfblk12/5(cfblk12)
  cfblk11/1(cfblk2) -> cfblk16/1, cfblk17/1, cfblk18/1
  cfblk4/1 -> cfblk3/1, cfblk11/3(cfblk11), cfblk6/3
  cfblk9/1(cfblk2) -> cfblk10/1(cfblk1), cfblk15/1, cfblk19/1
  cfblk13/1 -> cfblk11/1(cfblk1), cfblk12/4(cfblk11), cfblk10/3(cfblk7)
  cfblk6/1 -> cfblk9/3(cfblk16)
  cfblk5/1 -> cfblk11/2(cfblk10), cfblk11/4(cfblk12)
  cfblk1/1 -> cfblk12/1(cfblk1)
  cfblk3/1 -> cfblk6/2
  cfblk15/1 -> cfblk6/1
  cfblk16/1 -> cfblk9/2(cfblk15)
  cfblk17/1 -> cfblk12/2(cfblk9)
  cfblk18/1 -> cfblk12/3(cfblk10)
  cfblk19/1 -> cfblk3/2

== system sampleModel653/cfblk153 ==
  cfblk1 : Inport
  cfblk12 : Inport  Port=2
  cfblk13 : Inport  Port=3
  cfblk14 : Inport  Port=4
  cfblk15 : Inport  Port=5
  cfblk10 : Subsystem
  cfblk11 : Subsystem
  cfblk17 : Delay  SampleTime=1
  cfblk18 : Delay  SampleTime=1
  cfblk3 : simulink/Discrete/Tapped Delay  vinit=0.0  samptime=-1  NumDelays=1  DelayOrder=Oldest  includeCurrent=off
  cfblk4 : Sum  Inputs=+-
  cfblk5 : ComplexToRealImag
  cfblk6 : Constant  Value=[-310397297.897725]  SampleTime=1
  cfblk7 : Subsystem
  cfblk8 : Subsystem
  cfblk9 : Subsystem
  cfblk2 : Outport
  cfblk16 : Outport  Port=2
  wires:
  cfblk13/1 -> cfblk8/1(cfblk1)
  cfblk4/1 -> cfblk8/2(cfblk15)
  cfblk14/1 -> cfblk2/1
  cfblk6/1 -> cfblk4/1
  cfblk8/1(cfblk2) -> cfblk11/1(cfblk1)
  cfblk12/1 -> cfblk9/1(cfblk1)
  cfblk1/1 -> cfblk4/2
  cfblk11/1(cfblk2) -> cfblk16/1
  cfblk11/2(cfblk14) -> cfblk7/2(cfblk9)
  cfblk15/1 -> cfblk7/3(cfblk10)
  cfblk8/2(cfblk16) -> cfblk11/2(cfblk12)
  cfblk11/3(cfblk15) -> cfblk5/1
  cfblk5/1 -> cfblk9/2(cfblk11)
  cfblk5/2 -> cfblk9/3(cfblk12)
  cfblk8/3(cfblk17) -> cfblk10/1(cfblk1)
  cfblk7/1(cfblk2) -> cfblk9/4(cfblk13)
  cfblk7/2(cfblk11) -> cfblk3/1
  cfblk9/1(cfblk2) -> cfblk10/2(cfblk9)
  cfblk9/2(cfblk14) -> cfblk10/3(cfblk10)
  cfblk10/1(cfblk2) -> cfblk17/1
  cfblk17/1 -> cfblk11/3(cfblk13)
  cfblk3/1 -> cfblk18/1
  cfblk18/1 -> cfblk7/1(cfblk1)

== system sampleModel653/cfblk154 ==
  cfblk1 : Inport
  cfblk12 : Inport  Port=2
  cfblk13 : Inport  Port=3
  cfblk10 : Subsystem
  cfblk11 : Subsystem
  cfblk{14..17} (4 alike) : Delay  SampleTime=1
  cfblk3 : simulink/Discrete/Tapped Delay  vinit=0.0  samptime=-1  NumDelays=1  DelayOrder=Oldest  includeCurrent=off
  cfblk4 : DiscreteFir  SampleTime=1
  cfblk5 : simulink/Discrete/Tapped Delay  vinit=0.0  samptime=-1  NumDelays=1  DelayOrder=Oldest  includeCurrent=off
  cfblk6 : DiscreteIntegrator  ICPrevOutput=DiscIntNeverNeededParam  ICPrevScaledInput=DiscIntNeverNeededParam
  cfblk7 : Subsystem
  cfblk8 : Subsystem
  cfblk9 : Subsystem
  cfblk2 : Outport
  wires:
  cfblk11/1(cfblk2) -> cfblk8/1(cfblk1)
  cfblk8/1(cfblk2) -> cfblk4/1
  cfblk10/1(cfblk2) -> cfblk3/1
  cfblk11/2(cfblk11) -> cfblk9/1(cfblk1)
  cfblk8/2(cfblk8) -> cfblk10/1(cfblk1)
  cfblk1/1 -> cfblk5/1
  cfblk5/1 -> cfblk6/1
  cfblk12/1 -> cfblk11/2(cfblk7)
  cfblk6/1 -> cfblk11/3(cfblk8)
  cfblk9/2(cfblk7) -> cfblk2/1
  cfblk9/3(cfblk8) -> cfblk7/1(cfblk1)
  cfblk13/1 -> cfblk7/2(cfblk6)
  cfblk4/1 -> cfblk10/3(cfblk11)
  cfblk3/1 -> cfblk14/1
  cfblk14/1 -> cfblk10/2(cfblk10)
  cfblk8/3(cfblk9) -> cfblk15/1
  cfblk15/1 -> cfblk11/5(cfblk10)
  cfblk9/1(cfblk2) -> cfblk16/1
  cfblk16/1 -> cfblk11/1(cfblk1)
  cfblk7/1(cfblk2) -> cfblk17/1
  cfblk17/1 -> cfblk11/4(cfblk9)

== system sampleModel653/cfblk155 ==
  cfblk1 : Inport
  cfblk9 : Inport  Port=2
  cfblk{11..15} (5 alike) : Delay  SampleTime=1
  cfblk3 : simulink/Discrete/Transfer Fcn Real Zero  ZeroZ=0.75  ICPrevInput=0.0  DoSatur=off
  cfblk4 : Rounding
  cfblk5 : Constant  Value=[530424737.727567]  SampleTime=1
  cfblk6 : Subsystem
  cfblk7 : Subsystem
  cfblk8 : Subsystem
  cfblk2 : Outport
  cfblk10 : Outport  Port=2
  wires:
  cfblk1/1 -> cfblk7/1(cfblk1), cfblk6/2(cfblk10)
  cfblk5/1 -> cfblk3/1
  cfblk6/2(cfblk11) -> cfblk10/1
  cfblk3/1 -> cfblk2/1
  cfblk4/1 -> cfblk8/1(cfblk1), cfblk8/4(cfblk10)
  cfblk7/1(cfblk2) -> cfblk8/2(cfblk8)
  cfblk9/1 -> cfblk4/1, cfblk8/3(cfblk9)
  cfblk7/2(cfblk14) -> cfblk6/1(cfblk1)
  cfblk8/3(cfblk12) -> cfblk13/1, cfblk14/1
  cfblk8/1(cfblk2) -> cfblk11/1
  cfblk11/1 -> cfblk7/3(cfblk10)
  cfblk8/2(cfblk11) -> cfblk12/1
  cfblk12/1 -> cfblk7/4(cfblk11)
  cfblk13/1 -> cfblk7/5(cfblk12)
  cfblk14/1 -> cfblk7/6(cfblk13)
  cfblk6/1(cfblk2) -> cfblk15/1
  cfblk15/1 -> cfblk7/2(cfblk9)

== system sampleModel653/cfblk156 ==
  cfblk1 : Inport
  cfblk15 : Inport  Port=2
  cfblk10 : Subsystem
  cfblk11 : Subsystem
  cfblk12 : Subsystem
  cfblk13 : Subsystem
  cfblk14 : Subsystem
  cfblk{17..22} (6 alike) : Delay  SampleTime=1
  cfblk3 : DiscreteTransferFcn  SampleTime=1
  cfblk4 : DiscreteFir  SampleTime=1
  cfblk5 : Signum
  cfblk6 : Product
  cfblk7 : Polyval  Coefs=[ +2.081618890e-019, -1.441693666e-014, +4.719686976e-010, -8.536869453e-006, +1.621573104e-001, -8.087801117e+001 ]
  cfblk8 : Subsystem
  cfblk9 : Subsystem
  cfblk2 : Outport
  cfblk16 : Outport  Port=2
  wires:
  cfblk5/1 -> cfblk6/1, cfblk16/1, cfblk19/1
  cfblk4/1 -> cfblk3/1, cfblk14/3(cfblk10)
  cfblk15/1 -> cfblk12/1(cfblk1), cfblk10/2(cfblk10), cfblk11/4(cfblk7)
  cfblk12/1(cfblk2) -> cfblk9/1(cfblk1)
  cfblk1/1 -> cfblk11/1(cfblk1)
  cfblk14/1(cfblk2) -> cfblk5/1, cfblk12/4(cfblk13)
  cfblk11/1(cfblk2) -> cfblk8/1(cfblk1)
  cfblk13/1(cfblk2) -> cfblk4/1
  cfblk9/1(cfblk2) -> cfblk7/1
  cfblk13/2(cfblk14) -> cfblk6/2
  cfblk6/1 -> cfblk12/2(cfblk11)
  cfblk11/2(cfblk10) -> cfblk14/1(cfblk1), cfblk10/1(cfblk1)
  cfblk8/1(cfblk2) -> cfblk13/2(cfblk12)
  cfblk8/2(cfblk8) -> cfblk13/3(cfblk13), cfblk12/3(cfblk12), cfblk21/1
  cfblk10/2(cfblk11) -> cfblk14/2(cfblk9)
  cfblk10/3(cfblk12) -> cfblk2/1
  cfblk3/1 -> cfblk17/1
  cfblk17/1 -> cfblk8/2(cfblk7)
  cfblk7/1 -> cfblk18/1
  cfblk18/1 -> cfblk13/1(cfblk1)
  cfblk19/1 -> cfblk11/5(cfblk8)
  cfblk13/3(cfblk15) -> cfblk20/1
  cfblk20/1 -> cfblk11/3(cfblk6)
  cfblk21/1 -> cfblk11/6(cfblk9)
  cfblk10/1(cfblk2) -> cfblk22/1
  cfblk22/1 -> cfblk11/2(cfblk5)

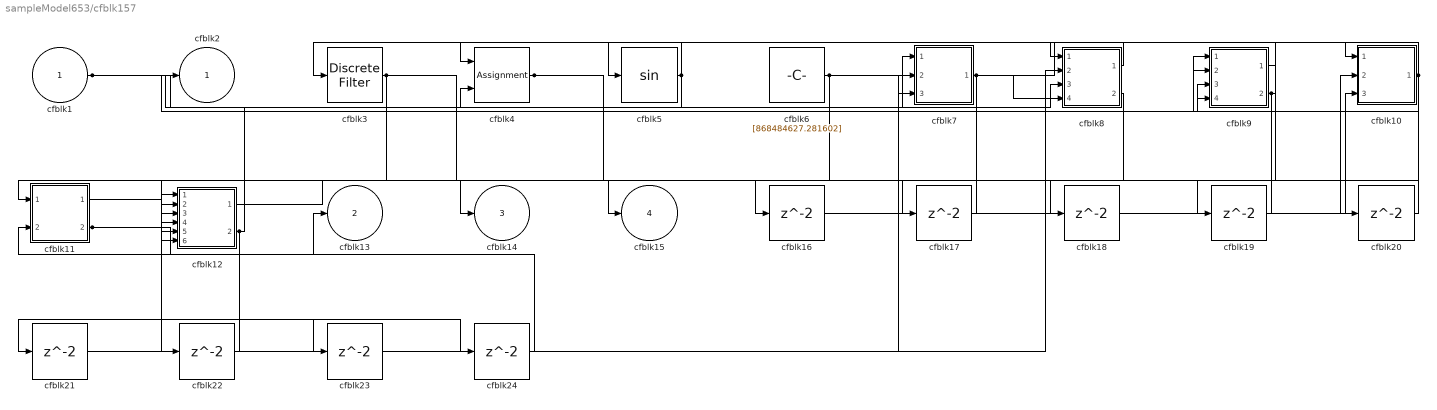
== system sampleModel653/cfblk157 ==
  cfblk1 : Inport
  cfblk10 : Subsystem
  cfblk11 : Subsystem
  cfblk12 : Subsystem
  cfblk{16..24} (9 alike) : Delay  SampleTime=1
  cfblk3 : DiscreteFilter  SampleTime=1
  cfblk4 : Assignment  DiagnosticForDimensions=Warning  IndexOptions=Index vector (dialog)  Indices=1  OutputSizes=1
  cfblk5 : Trigonometry
  cfblk6 : Constant  Value=[868484627.281602]  SampleTime=1
  cfblk7 : Subsystem
  cfblk8 : Subsystem
  cfblk9 : Subsystem
  cfblk2 : Outport
  cfblk13 : Outport  Port=2
  cfblk14 : Outport  Port=3
  cfblk15 : Outport  Port=4
  wires:
  cfblk8/1(cfblk2) -> cfblk3/1
  cfblk1/1 -> cfblk7/1(cfblk1), cfblk9/3(cfblk13)
  cfblk8/2(cfblk10) -> cfblk14/1
  cfblk10/1(cfblk2) -> cfblk15/1, cfblk5/1
  cfblk7/1(cfblk2) -> cfblk10/1(cfblk1), cfblk8/4(cfblk9), cfblk12/4(cfblk13), cfblk12/6(cfblk15)
  cfblk12/2(cfblk16) -> cfblk11/2(cfblk9), cfblk2/1, cfblk21/1
  cfblk4/1 -> cfblk9/4(cfblk14), cfblk16/1
  cfblk5/1 -> cfblk4/1, cfblk4/2
  cfblk9/2(cfblk15) -> cfblk8/1(cfblk1), cfblk12/5(cfblk14)
  cfblk6/1 -> cfblk11/1(cfblk1), cfblk8/3(cfblk8)
  cfblk3/1 -> cfblk12/3(cfblk12), cfblk18/1, cfblk19/1
  cfblk11/2(cfblk10) -> cfblk13/1, cfblk23/1, cfblk24/1
  cfblk16/1 -> cfblk10/2(cfblk14)
  cfblk9/1(cfblk2) -> cfblk17/1
  cfblk17/1 -> cfblk7/2(cfblk10)
  cfblk18/1 -> cfblk10/3(cfblk15)
  cfblk19/1 -> cfblk9/2(cfblk12)
  cfblk12/1(cfblk2) -> cfblk20/1
  cfblk20/1 -> cfblk9/1(cfblk1)
  cfblk21/1 -> cfblk7/3(cfblk11)
  cfblk11/1(cfblk2) -> cfblk22/1
  cfblk22/1 -> cfblk12/1(cfblk1)
  cfblk23/1 -> cfblk8/2(cfblk7)
  cfblk24/1 -> cfblk12/2(cfblk11)

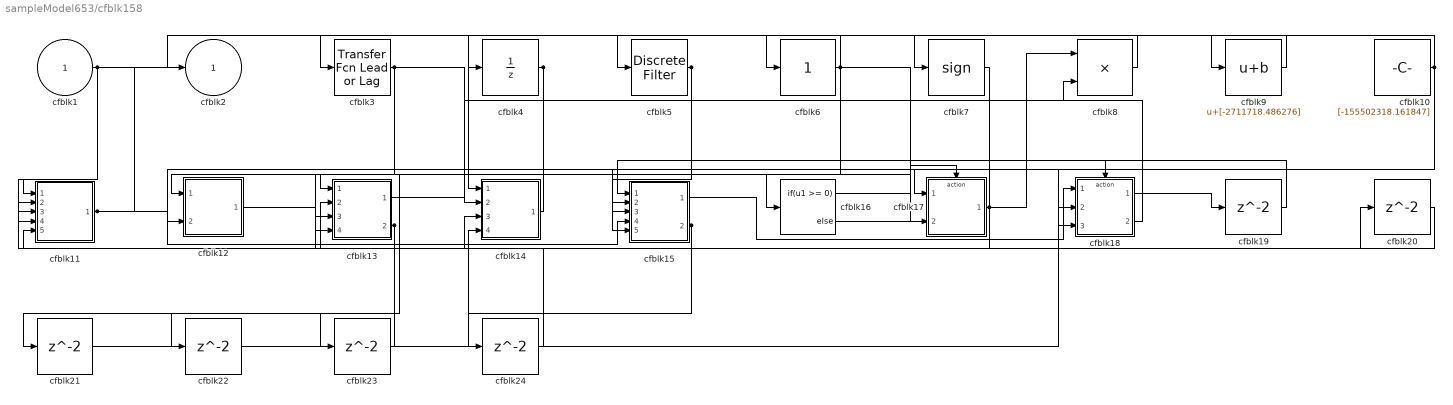
== system sampleModel653/cfblk158 ==
  cfblk1 : Inport
  cfblk10 : Constant  Value=[-155502318.161847]  SampleTime=1
  cfblk11 : Subsystem
  cfblk12 : Subsystem
  cfblk13 : Subsystem
  cfblk14 : Subsystem
  cfblk15 : Subsystem
  cfblk16 : If  IfExpression=u1 >= 0  SampleTime=1
  cfblk17 : Subsystem  TreatAsAtomicUnit=on
  cfblk18 : Subsystem  TreatAsAtomicUnit=on
  cfblk{19..24} (6 alike) : Delay  SampleTime=1
  cfblk3 : simulink/Discrete/Transfer Fcn Lead or Lag  PoleZ=0.95  ZeroZ=0.75  ICPrevOutput=0.0  ICPrevInput=0.0  DoSatur=off
  cfblk4 : UnitDelay  HasFrameUpgradeWarning=on
  cfblk5 : DiscreteFilter  SampleTime=1
  cfblk6 : simulink/Math Operations/Slider Gain  gain=1  low=0  high=2
  cfblk7 : Signum
  cfblk8 : Product  Inputs=**
  cfblk9 : Bias  Bias=[-2711718.486276]  SaturateOnIntegerOverflow=off
  cfblk2 : Outport
  wires:
  cfblk6/1 -> cfblk16/1, cfblk18/3(cfblk10), cfblk3/1, cfblk15/5(cfblk8)
  cfblk9/1 -> cfblk14/1(cfblk1)
  cfblk17/1(cfblk2) -> cfblk8/1, cfblk15/2(cfblk5), cfblk11/5(cfblk10)
  cfblk11/1(cfblk2) -> cfblk2/1, cfblk15/4(cfblk7)
  cfblk10/1 -> cfblk5/1, cfblk17/1(cfblk1)
  cfblk3/1 -> cfblk12/1(cfblk1), cfblk17/2(cfblk17)
  cfblk18/2(cfblk11) -> cfblk4/1
  cfblk13/1(cfblk2) -> cfblk8/2
  cfblk15/1(cfblk2) -> cfblk18/1(cfblk1)
  cfblk1/1 -> cfblk11/1(cfblk1), cfblk11/3(cfblk8), cfblk6/1, cfblk9/1
  cfblk7/1 -> cfblk12/2(cfblk8)
  cfblk13/2(cfblk13) -> cfblk21/1, cfblk22/1
  cfblk4/1 -> cfblk14/2(cfblk14), cfblk13/4(cfblk12), cfblk23/1
  cfblk14/1(cfblk2) -> cfblk13/1(cfblk1)
  cfblk8/1 -> cfblk7/1
  cfblk15/2(cfblk9) -> cfblk13/2(cfblk10), cfblk24/1
  cfblk5/1 -> cfblk13/3(cfblk11), cfblk15/3(cfblk6)
  cfblk16/1 -> cfblk17/Action
  cfblk16/2 -> cfblk18/Action
  cfblk18/1(cfblk2) -> cfblk19/1
  cfblk19/1 -> cfblk15/1(cfblk1)
  cfblk12/1(cfblk2) -> cfblk20/1
  cfblk20/1 -> cfblk14/3(cfblk15)
  cfblk21/1 -> cfblk18/2(cfblk9)
  cfblk22/1 -> cfblk14/4(cfblk16)
  cfblk23/1 -> cfblk11/4(cfblk9)
  cfblk24/1 -> cfblk11/2(cfblk7)

== system sampleModel653/cfblk159 ==
  cfblk1 : Inport
  cfblk6 : Inport  Port=2
  cfblk3 : DiscreteIntegrator  ICPrevOutput=DiscIntNeverNeededParam  ICPrevScaledInput=DiscIntNeverNeededParam
  cfblk4 : Sum  Inputs=+-
  cfblk5 : UnaryMinus
  cfblk2 : Outport
  cfblk7 : Outport  Port=2
  cfblk8 : Outport  Port=3
  wires:
  cfblk1/1 -> cfblk7/1, cfblk4/1
  cfblk3/1 -> cfblk5/1
  cfblk5/1 -> cfblk8/1
  cfblk6/1 -> cfblk3/1, cfblk4/2
  cfblk4/1 -> cfblk2/1

== system sampleModel653/cfblk160 ==
  cfblk1 : Inport
  cfblk8 : Inport  Port=2
  cfblk10 : Delay  SampleTime=1
  cfblk3 : DiscreteFilter  SampleTime=1
  cfblk4 : Constant  Value=[-272270658.444751]  SampleTime=1
  cfblk5 : Subsystem
  cfblk6 : Subsystem
  cfblk7 : Subsystem
  cfblk2 : Outport
  cfblk9 : Outport  Port=2
  wires:
  cfblk8/1 -> cfblk3/1, cfblk5/3(cfblk14)
  cfblk3/1 -> cfblk7/1(cfblk1)
  cfblk5/1(cfblk2) -> cfblk6/1(cfblk1)
  cfblk6/1(cfblk2) -> cfblk9/1
  cfblk4/1 -> cfblk6/2(cfblk8)
  cfblk7/1(cfblk2) -> cfblk2/1
  cfblk1/1 -> cfblk5/1(cfblk1)
  cfblk6/2(cfblk9) -> cfblk7/2(cfblk7)
  cfblk6/3(cfblk10) -> cfblk10/1
  cfblk10/1 -> cfblk5/2(cfblk13)
